simulink model "FIR"  (R2020a)
settings: Solver=VariableStepAuto  StartTime=0.0  StopTime=0.01  RelTol=1e-3
libraries: xbsIndex_r4 x5, dspfdesign x1
settings Model: Creator=Lenovo  LastModifiedBy=Lenovo

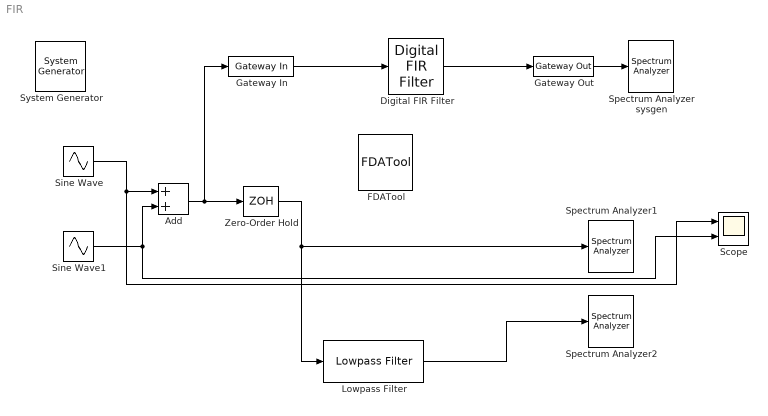
== system FIR ==
  " System Generator" : xbsIndex_r4/ System Generator  Tag=genX  xilinxfamily=zynq  part=xc7z020  speed=-1  package=clg484  synthesis_tool=Vivado  clock_wrapper=Clock Enables  directory=./netlist  proj_type=Vivado  Synth_file=Vivado Synthesis Defaults  Impl_file=Vivado Implementation Defaults  testbench=off  simulink_period=1/20e6  sysclk_period=50  dcm_input_clock_period=10  incr_netlist=off  trim_vbits=Everywhere in SubSystem  dbl_ovrd=According to Block Masks  core_generation=According to Block Masks  run_coregen=off  deprecated_control=off  eval_field=0  block_type=sysgen
  Add : Sum
  Digital FIR Filter : xbsIndex_r4/Digital FIR Filter  coeff_source=off  coefficientvector=fir1(15,0.5)  coeff_calulate=on  coefficient_width=11  coefficient_fractional_bits=11  interpolation_filter_rate=1  decimation_filter_rate=1  fda_coefficientvector=[0.00775647470182829 -1.42922362923963e-05 -0.0538933995947213 4.30114467150759e-05 0.296165761405981 0.499940603924084 0.296165761405981 4.30114467150759e-05 -0.0538933995947213 -1.42922362923963e-05 0.00775647470182829]  simulation_type=fast_sim  simulation_model=sysgen:fir_macro  block_type=fir_macro
  FDATool : xbsIndex_r4/FDATool  block_type=fdatool
      settings: infoedit=FDATool
  Gateway In : xbsIndex_r4/Gateway In  gui_display_data_type=Fixed-point  arith_type="Signed  (2's comp)"  n_bits=16  bin_pt=14  preci_type=Single  exp_width=8  frac_width=24  rows=1  columns=1  quantization="Round  (unbiased: +/- Inf)"  overflow=Saturate  period=1/20e6  UseAsADC=off  ADCChannel='1'  interface=None  automatic_assignment=on  address_offset=hex2dec('00')  intf_name=''  intf_description=''  default_value=0  timing_constraint=None  locs_specified=off  LOCs={}  io_standard={}  inherit_from_input=off  hdl_port=on  dbl_ovrd=off  block_type=gatewayin
  Gateway Out : xbsIndex_r4/Gateway Out  inherit_from_input=off  hdl_port=on  rows=1  columns=1  UseAsDAC=off  DACChannel='1'  interface=None  automatic_assignment=on  address_offset=hex2dec('00')  intf_name=''  intf_description=''  timing_constraint=None  locs_specified=off  LOCs={}  io_standard={}  block_type=gatewayout
  Lowpass Filter : dspfdesign/Lowpass Filter  FilterType=FIR  DesignForMinimumOrder=on  FilterOrder=50  PassbandFrequency=1.5e6  StopbandFrequency=8.5e6  PassbandRipple=0.01  StopbandAttenuation=80  InheritSampleRate=off  SampleRate=20e6  SimulateUsing=Interpreted execution  roundingMode=Floor  coeffsDataTypeStr=fixdt(1,16)
  Scope : Scope  NumInputPorts=2
  Sine Wave : Sin  Frequency=2*pi*9e6  SampleTime=0
  Sine Wave1 : Sin  Frequency=2*pi*1e6  SampleTime=0
  Spectrum Analyzer sysgen : SpectrumAnalyzer
  Spectrum Analyzer1 : SpectrumAnalyzer
  Spectrum Analyzer2 : SpectrumAnalyzer
  Zero-Order Hold : ZeroOrderHold  SampleTime=1/20e6
  wires:
  Sine Wave/1 -> Scope/1, Add/1
  Sine Wave1/1 -> Add/2, Scope/2
  Add/1 -> Gateway In/1, Zero-Order Hold/1
  Zero-Order Hold/1 -> Spectrum Analyzer1/1, Lowpass Filter/1
  Lowpass Filter/1 -> Spectrum Analyzer2/1
  Gateway In/1 -> Digital FIR Filter/1
  Digital FIR Filter/1 -> Gateway Out/1
  Gateway Out/1 -> Spectrum Analyzer sysgen/1
